simulink model "CerebellumIODCNAbstractFext"  (Simulink 7.4)
settings: Solver=ode3  StartTime=0.0  StopTime=1.  FixedStep=0.002  RelTol=1e-3
values from neighbouring files (symbols this model uses):
  RRedKuKa = RRedKuKa    [LaunchCerebellumSimulink.m]    (also in LaunchCerebellumSimulinkExternalForce.m; MANIPULATORS.mat = )
undefined symbols (not defined in the file or in its folder): frne
libraries: simulink x1
(part 1 of 2)
settings Model: Creator=Sensopac  LastModifiedBy=Sensopac
settings SimEventsCC: propDiagAttribOutput=1  propDiagFcnCallOutput=1  propDiagStatOutput=0

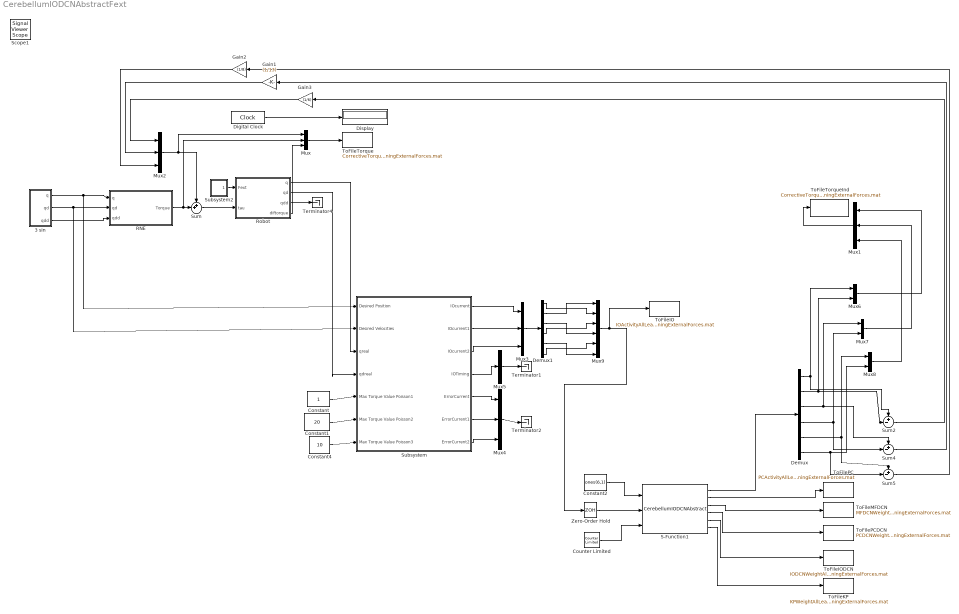
== system CerebellumIODCNAbstractFext ==
  3 sin : Subsystem
  Constant : Constant  OutDataType=sfix(16)  OutScaling=2^0
  Constant1 : Constant  Value=20  OutDataType=sfix(16)  OutScaling=2^0
  Constant2 : Constant  Value=ones(6,1)  OutDataTypeMode=double  OutDataType=sfix(16)  OutScaling=2^0  OutDataTypeStr=double  SampleTime=0.002
  Constant4 : Constant  Value=10  OutDataType=sfix(16)  OutScaling=2^0
  Counter Limited : simulink/Sources/Counter Limited  SystemSampleTime=-1  uplimit=499  tsamp=0.002
  Demux : Demux  Outputs=6
  Demux1 : Demux  Outputs=6
  Digital Clock : DigitalClock  SampleTime=0.002
  Display : Display
  Gain1 : Gain  Gain=(1/13)  ParameterDataType=fixdt(1, 16)  ParameterScaling=2^0  OutDataType=fixdt(1, 16)  OutScaling=2^0
  Gain2 : Gain  Gain=(1/8)  ParameterDataType=fixdt(1, 16)  ParameterScaling=2^0  OutDataType=fixdt(1, 16)  OutScaling=2^0
  Gain3 : Gain  Gain=(1/6)  ParameterDataType=fixdt(1, 16)  ParameterScaling=2^0  OutDataType=fixdt(1, 16)  OutScaling=2^0
  Mux{,1..4} (5 alike) : Mux  Inputs=3
  Mux5 : Mux  Inputs=1
  Mux6 : Mux  Inputs=2
  Mux7 : Mux  Inputs=2
  Mux8 : Mux  Inputs=2
  Mux9 : Mux  Inputs=6
  "RNE " : Subsystem  mask{grav=[ 0 0 9.81], RRed=RRedKuKa}
      mask prompts: grav "Gravity Vector( 0 0  -9.81)"; RRed "Robot"
      mask help:
      | This block computes the inverse dynamics by using the
      | recursive Newton Euler algorithm(computationally speaking more efficient than Lagrange-Euler's method)
      | The gravity vector has to be set (the gravity direction has to be taken into account)
      mask Display:
      | port_label('output',1,'Torques')
      | port_label('input',1,'q')
      | port_label('input',2,'qd')
      | port_label('input',3,'qdd')
      | fprintf('RNE')
  Robot : Subsystem
  S-Function1 : S-Function  FunctionName=CerebellumIODCNAbstract  Parameters=ParamFile NumberOfJoints NumberOfStates WeightFile  EnableBusSupport=off  mask{ParamFile='Parameters.txt', NumberOfJoints=6, NumberOfStates=500, WeightFile='./Register/WeightsNF.dat'}
      mask prompts: ParamFile "Learning Configuration File"; NumberOfJoints "Number Of Joints"; NumberOfStates "Number Of States"; WeightFile "Final Weight File"
      mask Display:
      | image(imread('EDLUTIcon.jpg'));
      | port_label('input',1,'MFAct')
      | port_label('input',2,'Error')
      | port_label('input',3,'State')
      | port_label('output',1,'DCNAct')
      | port_label('output',2,'PCAct')
      | port_label('output',3,'MFWeight')
      | port_label('output',4,'PCWeight')
      | port_label('output',5,'IOWeight')
      | port_label('output',6,'KPWeight')
      | fprintf('Cerebellum')
  Subsystem : Subsystem
  Subsystem2 : Subsystem
  Sum : Sum  Inputs=++|  OutDataType=sfix(16)  OutScaling=2^0
  Sum2 : Sum  Inputs=+-|  OutDataType=sfix(16)  OutScaling=2^0
  Sum4 : Sum  Inputs=+-|  OutDataType=sfix(16)  OutScaling=2^0
  Sum5 : Sum  Inputs=+-|  OutDataType=sfix(16)  OutScaling=2^0
  Terminator1 : Terminator
  Terminator2 : Terminator
  Terminator4 : Terminator
  ToFileIO : ToFile  Filename=IOActivityAllLearningExternalForces.mat
  ToFileIODCN : ToFile  Filename=IODCNWeightAllLearningExternalForces.mat
  ToFileKP : ToFile  Filename=KPWeightAllLearningExternalForces.mat
  ToFileMFDCN : ToFile  Filename=MFDCNWeightAllLearningExternalForces.mat
  ToFilePC : ToFile  Filename=PCActivityAllLearningExternalForces.mat
  ToFilePCDCN : ToFile  Filename=PCDCNWeightAllLearningExternalForces.mat
  ToFileTorque : ToFile  Filename=CorrectiveTorqueAllLearningExternalForces.mat
  ToFileTorqueInd : ToFile  Filename=CorrectiveTorque1AllLearningExternalForces.mat
  Zero-Order Hold : ZeroOrderHold  SampleTime=0.002
  Scope1 : SignalViewerScope  IOType=viewer  RefreshTime=0.035000
  wires:
  3 sin/1(q) -> Subsystem/1(Desired Position), "RNE "/1(q)
  3 sin/2(qd) -> Subsystem/2(Desired Velocities), "RNE "/2(qd)
  3 sin/3(qdd) -> "RNE "/3(qdd)
  "RNE "/1(Torque) -> Sum/2, Mux/2
  Robot/1(q) -> Subsystem/3(qreal)
  Robot/2(qd) -> Subsystem/4(qdreal)
  Sum/1 -> Robot/2(tau)
  Robot/3(qdd) -> Terminator4/1
  Mux2/1 -> Mux/1, Sum/1
  Mux/1 -> ToFileTorque/1
  Mux1/1 -> ToFileTorqueInd/1
  Counter Limited/1 -> S-Function1/3
  Constant2/1 -> S-Function1/1
  S-Function1/1 -> Demux/1
  S-Function1/2 -> ToFilePC/1
  S-Function1/3 -> ToFileMFDCN/1
  S-Function1/4 -> ToFilePCDCN/1
  Zero-Order Hold/1 -> S-Function1/2
  Mux6/1 -> Mux1/1
  Mux7/1 -> Mux1/2
  Mux8/1 -> Mux1/3
  Demux/1 -> Sum2/1, Mux6/1
  Demux/3 -> Sum4/1, Mux7/1
  Demux/5 -> Sum5/1, Mux8/1
  Demux/6 -> Sum5/2, Mux8/2
  Demux/4 -> Sum4/2, Mux7/2
  Demux/2 -> Sum2/2, Mux6/2
  Sum2/1 -> Gain3/1
  Sum4/1 -> Gain1/1
  Sum5/1 -> Gain2/1
  Mux5/1 -> Terminator1/1
  Mux4/1 -> Terminator2/1
  Subsystem/4(IOTiming) -> Mux5/1
  Subsystem/5(ErrorCurrent) -> Mux4/1
  Subsystem/6(ErrorCurrent1) -> Mux4/2
  Subsystem/7(ErrorCurrent2) -> Mux4/3
  Mux3/1 -> Demux1/1
  Mux9/1 -> ToFileIO/1, Zero-Order Hold/1
  Demux1/2 -> Mux9/1
  Demux1/1 -> Mux9/2
  Demux1/3 -> Mux9/4
  Demux1/4 -> Mux9/3
  Demux1/5 -> Mux9/6
  Demux1/6 -> Mux9/5
  Subsystem/1(IOcurrent) -> Mux3/1
  Subsystem/2(IOcurrent1) -> Mux3/2
  Subsystem/3(IOcurrent2) -> Mux3/3
  Digital Clock/1 -> Display/1
  Gain2/1 -> Mux2/3
  Gain1/1 -> Mux2/2
  Gain3/1 -> Mux2/1
  S-Function1/5 -> ToFileIODCN/1
  S-Function1/6 -> ToFileKP/1
  Subsystem2/1(Fx,y,z) -> Robot/1(Fext)
  Robot/4(diftorque) -> Mux/3
  Constant/1 -> Subsystem/5(" Max Torque Value Poisson1")
  Constant1/1 -> Subsystem/6(" Max Torque Value Poisson2")
  Constant4/1 -> Subsystem/7(" Max Torque Value Poisson3")

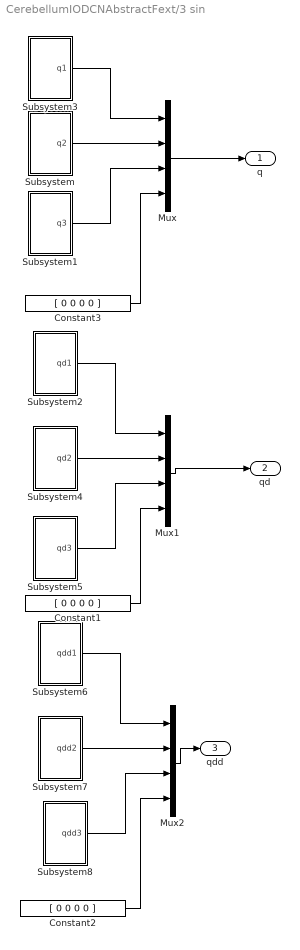
== system CerebellumIODCNAbstractFext/3 sin ==
  Constant1 : Constant  Value=[ 0 0 0 0 ]  OutDataType=sfix(16)  OutScaling=2^0
  Constant2 : Constant  Value=[ 0 0 0 0 ]  OutDataType=sfix(16)  OutScaling=2^0
  Constant3 : Constant  Value=[ 0 0 0 0 ]  OutDataType=sfix(16)  OutScaling=2^0
  Mux : Mux
  Mux1 : Mux
  Mux2 : Mux
  Subsystem : Subsystem
  Subsystem1 : Subsystem
  Subsystem2 : Subsystem
  Subsystem3 : Subsystem
  Subsystem4 : Subsystem
  Subsystem5 : Subsystem
  Subsystem6 : Subsystem
  Subsystem7 : Subsystem
  Subsystem8 : Subsystem
  q : Outport  OutDataType=sfix(16)  OutScaling=2^0
  qd : Outport  Port=2  OutDataType=sfix(16)  OutScaling=2^0
  qdd : Outport  Port=3  OutDataType=sfix(16)  OutScaling=2^0
  wires:
  Mux2/1 -> qdd/1
  Mux1/1 -> qd/1
  Mux/1 -> q/1
  Subsystem3/1(q1) -> Mux/1
  Subsystem/1(q2) -> Mux/2
  Subsystem1/1(q3) -> Mux/3
  Subsystem2/1(qd1) -> Mux1/1
  Subsystem4/1(qd2) -> Mux1/2
  Subsystem5/1(qd3) -> Mux1/3
  Subsystem6/1(qdd1) -> Mux2/1
  Subsystem7/1(qdd2) -> Mux2/2
  Subsystem8/1(qdd3) -> Mux2/3
  Constant3/1 -> Mux/4
  Constant1/1 -> Mux1/4
  Constant2/1 -> Mux2/4

== system CerebellumIODCNAbstractFext/RNE  ==
  q : Inport  OutDataType=sfix(16)  OutScaling=2^0
  qd : Inport  Port=2  OutDataType=sfix(16)  OutScaling=2^0
  qdd : Inport  Port=3  OutDataType=sfix(16)  OutScaling=2^0
  Mux : Mux  Inputs=3
  S-Function : S-Function  FunctionName=Select  Parameters=RRed  EnableBusSupport=off
  S-Function1 : S-Function  FunctionName=Select  Parameters=RRed  EnableBusSupport=off
  S-Function2 : S-Function  FunctionName=Select  Parameters=RRed  EnableBusSupport=off
  rne : MATLABFcn  MATLABFcn=frne(RRed, u(1:RRed.n)', u(RRed.n+1:2*RRed.n)', u(2* RRed.n+1:3*RRed.n)',grav)  OutputDimensions=RRed.n
  Torque : Outport  OutDataType=sfix(16)  OutScaling=2^0
  wires:
  qdd/1 -> S-Function2/1
  rne/1 -> Torque/1
  q/1 -> S-Function/1
  Mux/1 -> rne/1
  qd/1 -> S-Function1/1
  S-Function/1 -> Mux/1
  S-Function1/1 -> Mux/2
  S-Function2/1 -> Mux/3

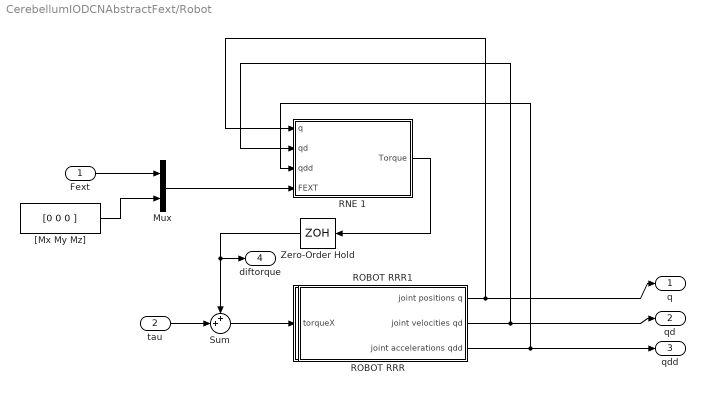
== system CerebellumIODCNAbstractFext/Robot ==
  Fext : Inport  OutDataType=sfix(16)  OutScaling=2^0
  tau : Inport  Port=2  OutDataType=sfix(16)  OutScaling=2^0
  Mux : Mux  Inputs=2
  RNE 1 : Subsystem  mask{grav=[ 0 0 9.81], RRed=RRedKuKa}
      mask prompts: grav "Gravity Vector ( 0 0  -9.81)"; RRed "Robot"
      mask help:
      | This block computes the inverse dynamics by using the
      | recursive Newton Euler algorithm(computationally speaking more efficient than Lagrange-Euler's method)
      | The gravity vector has to be set (the gravity direction has to be taken into account)
      mask Display:
      | port_label('output',1,'Torque')
      | port_label('input',1,'q')
      | port_label('input',2,'qd')
      | port_label('input',3,'qdd')
      | port_label('input',4,'Fext')
      | fprintf('RNE')
  ROBOT RRR : Subsystem  mask{Ciniciales=[0.0  0.1*sin(pi/4)  0.1 0 0 0 0], Viniciales=[2*pi*0.1 2*pi*sin(pi/4)*0.1 0 0 0 0 0], RRed=RRedKuKa}
      mask prompts: Ciniciales "Position initial conditions q"; Viniciales "Velocity initial conditions qd"; RRed "Robot"
      mask help: Simulated robot model(Rigid body dynamics)
  ROBOT RRR1 : Subsystem  mask{Ciniciales=[0.0  0.1*sin(pi/4)  0.1 0 0 0 0], Viniciales=[2*pi*0.1 2*pi*sin(pi/4)*0.1 0 0 0 0 0], RRed=RRedKuKa}
      mask prompts: Ciniciales "Position initial conditions q"; Viniciales "Velocity initial conditions qd"; RRed "Robot"
      mask help: Simulated robot model(Rigid body dynamics)
  Sum : Sum  Inputs=++|  OutDataType=sfix(16)  OutScaling=2^0
  Zero-Order Hold : ZeroOrderHold  SampleTime=0.002
  "[Mx My Mz]" : Constant  Value=[0 0 0 ]  OutDataType=sfix(16)  OutScaling=2^0
  q : Outport  OutDataType=sfix(16)  OutScaling=2^0
  qd : Outport  Port=2  OutDataType=sfix(16)  OutScaling=2^0
  qdd : Outport  Port=3  OutDataType=sfix(16)  OutScaling=2^0
  diftorque : Outport  Port=4  OutDataType=sfix(16)  OutScaling=2^0
  wires:
  ROBOT RRR/1(joint positions q) -> q/1, RNE 1/1(q)
  ROBOT RRR/2(joint velocities qd) -> qd/1, RNE 1/2(qd)
  ROBOT RRR/3(joint accelerations qdd) -> qdd/1, RNE 1/3(qdd)
  tau/1 -> Sum/2
  "[Mx My Mz]"/1 -> Mux/2
  Fext/1 -> Mux/1
  Mux/1 -> RNE 1/4(FEXT)
  RNE 1/1(Torque) -> Zero-Order Hold/1
  Sum/1 -> ROBOT RRR/1(torqueX)
  Zero-Order Hold/1 -> Sum/1, diftorque/1

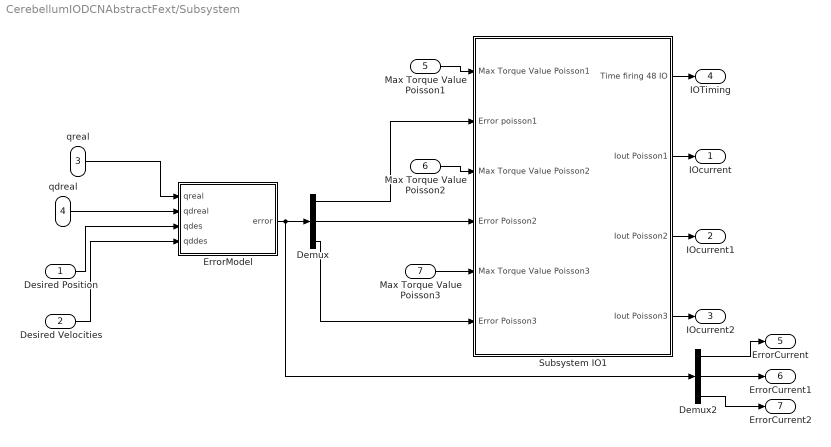
== system CerebellumIODCNAbstractFext/Subsystem ==
  Desired Position : Inport
  Desired Velocities : Inport  Port=2
  qreal : Inport  Port=3  OutDataType=sfix(16)  OutScaling=2^0
  qdreal : Inport  Port=4  OutDataType=sfix(16)  OutScaling=2^0
  " Max Torque Value Poisson1" : Inport  Port=5  OutDataType=sfix(16)  OutScaling=2^0
  " Max Torque Value Poisson2" : Inport  Port=6  OutDataType=sfix(16)  OutScaling=2^0
  " Max Torque Value Poisson3" : Inport  Port=7  OutDataType=sfix(16)  OutScaling=2^0
  Demux : Demux  Outputs=3
  Demux2 : Demux  Outputs=3
  ErrorModel : Subsystem
  Subsystem IO1 : Subsystem
  IOcurrent : Outport
  IOcurrent1 : Outport  Port=2
  IOcurrent2 : Outport  Port=3
  IOTiming : Outport  Port=4
  ErrorCurrent : Outport  Port=5
  ErrorCurrent1 : Outport  Port=6
  ErrorCurrent2 : Outport  Port=7
  wires:
  Desired Position/1 -> ErrorModel/3(qdes)
  Desired Velocities/1 -> ErrorModel/4(qddes)
  Subsystem IO1/1(Time firing 48 IO) -> IOTiming/1
  Demux/1 -> Subsystem IO1/2(Error poisson1)
  Subsystem IO1/2(Iout Poisson1) -> IOcurrent/1
  Demux/2 -> Subsystem IO1/4(Error Poisson2)
  Subsystem IO1/3(Iout Poisson2) -> IOcurrent1/1
  Demux/3 -> Subsystem IO1/6(Error Poisson3)
  Subsystem IO1/4(Iout Poisson3) -> IOcurrent2/1
  ErrorModel/1(error) -> Demux/1, Demux2/1
  qreal/1 -> ErrorModel/1(qreal)
  qdreal/1 -> ErrorModel/2(qdreal)
  Demux2/1 -> ErrorCurrent/1
  Demux2/2 -> ErrorCurrent1/1
  Demux2/3 -> ErrorCurrent2/1
  " Max Torque Value Poisson1"/1 -> Subsystem IO1/1(" Max Torque Value Poisson1")
  " Max Torque Value Poisson2"/1 -> Subsystem IO1/3(" Max Torque Value Poisson2")
  " Max Torque Value Poisson3"/1 -> Subsystem IO1/5(" Max Torque Value Poisson3")

== system CerebellumIODCNAbstractFext/Subsystem2 ==
  Mux : Mux  Inputs=3
  Subsystem : Subsystem
  Subsystem1 : Subsystem
  Subsystem3 : Subsystem
  Fx,y,z : Outport  OutDataType=sfix(16)  OutScaling=2^0
  wires:
  Mux/1 -> Fx,y,z/1
  Subsystem3/1(q1) -> Mux/1
  Subsystem/1(q2) -> Mux/2
  Subsystem1/1(q3) -> Mux/3

== system CerebellumIODCNAbstractFext/3 sin/Subsystem ==
  Constant1 : Constant  Value=0.1  OutDataType=sfix(16)  OutScaling=2^0
  Constant2 : Constant  Value=pi/4  OutDataType=sfix(16)  OutScaling=2^0
  Constant3 : Constant  Value=2*pi  OutDataType=sfix(16)  OutScaling=2^0
  Digital Clock : DigitalClock  SampleTime=0.002
  Product : Product  OutDataType=sfix(16)  OutScaling=2^0  RndMeth=Zero
  Product2 : Product  OutDataType=sfix(16)  OutScaling=2^0  RndMeth=Zero
  Sum : Sum  Inputs=|++  OutDataType=sfix(16)  OutScaling=2^0
  Trigonometric Function : Trigonometry
  q2 : Outport  OutDataType=sfix(16)  OutScaling=2^0
  wires:
  Sum/1 -> Trigonometric Function/1
  Constant2/1 -> Sum/1
  Product2/1 -> Sum/2
  Product/1 -> q2/1
  Trigonometric Function/1 -> Product/2
  Constant3/1 -> Product2/1
  Digital Clock/1 -> Product2/2
  Constant1/1 -> Product/1

== system CerebellumIODCNAbstractFext/3 sin/Subsystem1 ==
  Constant2 : Constant  Value=0.1  OutDataType=sfix(16)  OutScaling=2^0
  Constant3 : Constant  Value=pi/2  OutDataType=sfix(16)  OutScaling=2^0
  Constant4 : Constant  Value=2*pi  OutDataType=sfix(16)  OutScaling=2^0
  Digital Clock : DigitalClock  SampleTime=0.002
  Product : Product  OutDataType=sfix(16)  OutScaling=2^0  RndMeth=Zero
  Product2 : Product  OutDataType=sfix(16)  OutScaling=2^0  RndMeth=Zero
  Sum : Sum  Inputs=|++  OutDataType=sfix(16)  OutScaling=2^0
  Trigonometric Function : Trigonometry
  q3 : Outport  OutDataType=sfix(16)  OutScaling=2^0
  wires:
  Sum/1 -> Trigonometric Function/1
  Constant3/1 -> Sum/1
  Product2/1 -> Sum/2
  Product/1 -> q3/1
  Trigonometric Function/1 -> Product/2
  Constant4/1 -> Product2/1
  Digital Clock/1 -> Product2/2
  Constant2/1 -> Product/1

== system CerebellumIODCNAbstractFext/3 sin/Subsystem2 ==
  Constant1 : Constant  Value=0.1*2*pi  OutDataType=sfix(16)  OutScaling=2^0
  Constant3 : Constant  Value=2*pi  OutDataType=sfix(16)  OutScaling=2^0
  Digital Clock : DigitalClock  SampleTime=0.002
  Product : Product  OutDataType=sfix(16)  OutScaling=2^0  RndMeth=Zero
  Product2 : Product  OutDataType=sfix(16)  OutScaling=2^0  RndMeth=Zero
  Trigonometric Function : Trigonometry  Operator=cos
  qd1 : Outport  OutDataType=sfix(16)  OutScaling=2^0
  wires:
  Product/1 -> qd1/1
  Trigonometric Function/1 -> Product/2
  Constant3/1 -> Product2/1
  Product2/1 -> Trigonometric Function/1
  Digital Clock/1 -> Product2/2
  Constant1/1 -> Product/1

== system CerebellumIODCNAbstractFext/3 sin/Subsystem3 ==
  Constant1 : Constant  Value=0.1  OutDataType=sfix(16)  OutScaling=2^0
  Constant3 : Constant  Value=2*pi  OutDataType=sfix(16)  OutScaling=2^0
  Digital Clock : DigitalClock  SampleTime=0.002
  Product : Product  OutDataType=sfix(16)  OutScaling=2^0  RndMeth=Zero
  Product2 : Product  OutDataType=sfix(16)  OutScaling=2^0  RndMeth=Zero
  Trigonometric Function : Trigonometry
  q1 : Outport  OutDataType=sfix(16)  OutScaling=2^0
  wires:
  Product/1 -> q1/1
  Trigonometric Function/1 -> Product/2
  Constant3/1 -> Product2/1
  Product2/1 -> Trigonometric Function/1
  Digital Clock/1 -> Product2/2
  Constant1/1 -> Product/1

== system CerebellumIODCNAbstractFext/3 sin/Subsystem4 ==
  Constant1 : Constant  Value=0.1*2*pi  OutDataType=sfix(16)  OutScaling=2^0
  Constant2 : Constant  Value=pi/4  OutDataType=sfix(16)  OutScaling=2^0
  Constant3 : Constant  Value=2*pi  OutDataType=sfix(16)  OutScaling=2^0
  Digital Clock : DigitalClock  SampleTime=0.002
  Product : Product  OutDataType=sfix(16)  OutScaling=2^0  RndMeth=Zero
  Product2 : Product  OutDataType=sfix(16)  OutScaling=2^0  RndMeth=Zero
  Sum : Sum  Inputs=|++  OutDataType=sfix(16)  OutScaling=2^0
  Trigonometric Function : Trigonometry  Operator=cos
  qd2 : Outport  OutDataType=sfix(16)  OutScaling=2^0
  wires:
  Sum/1 -> Trigonometric Function/1
  Constant2/1 -> Sum/1
  Product2/1 -> Sum/2
  Product/1 -> qd2/1
  Trigonometric Function/1 -> Product/2
  Constant3/1 -> Product2/1
  Digital Clock/1 -> Product2/2
  Constant1/1 -> Product/1

== system CerebellumIODCNAbstractFext/3 sin/Subsystem5 ==
  Constant1 : Constant  Value=0.1*2*pi  OutDataType=sfix(16)  OutScaling=2^0
  Constant3 : Constant  Value=pi/2  OutDataType=sfix(16)  OutScaling=2^0
  Constant4 : Constant  Value=2*pi  OutDataType=sfix(16)  OutScaling=2^0
  Digital Clock : DigitalClock  SampleTime=0.002
  Product : Product  OutDataType=sfix(16)  OutScaling=2^0  RndMeth=Zero
  Product2 : Product  OutDataType=sfix(16)  OutScaling=2^0  RndMeth=Zero
  Sum : Sum  Inputs=|++  OutDataType=sfix(16)  OutScaling=2^0
  Trigonometric Function : Trigonometry  Operator=cos
  qd3 : Outport  OutDataType=sfix(16)  OutScaling=2^0
  wires:
  Sum/1 -> Trigonometric Function/1
  Constant3/1 -> Sum/1
  Product2/1 -> Sum/2
  Product/1 -> qd3/1
  Trigonometric Function/1 -> Product/2
  Constant4/1 -> Product2/1
  Digital Clock/1 -> Product2/2
  Constant1/1 -> Product/1

== system CerebellumIODCNAbstractFext/3 sin/Subsystem6 ==
  Constant1 : Constant  Value=-0.1*4*pi^2  OutDataType=sfix(16)  OutScaling=2^0
  Constant3 : Constant  Value=2*pi  OutDataType=sfix(16)  OutScaling=2^0
  Digital Clock : DigitalClock  SampleTime=0.002
  Product : Product  OutDataType=sfix(16)  OutScaling=2^0  RndMeth=Zero
  Product2 : Product  OutDataType=sfix(16)  OutScaling=2^0  RndMeth=Zero
  Trigonometric Function : Trigonometry
  qdd1 : Outport  OutDataType=sfix(16)  OutScaling=2^0
  wires:
  Product/1 -> qdd1/1
  Trigonometric Function/1 -> Product/2
  Constant3/1 -> Product2/1
  Product2/1 -> Trigonometric Function/1
  Digital Clock/1 -> Product2/2
  Constant1/1 -> Product/1

== system CerebellumIODCNAbstractFext/3 sin/Subsystem7 ==
  Constant1 : Constant  Value=-0.1*4*pi^2  OutDataType=sfix(16)  OutScaling=2^0
  Constant2 : Constant  Value=pi/4  OutDataType=sfix(16)  OutScaling=2^0
  Constant3 : Constant  Value=2*pi  OutDataType=sfix(16)  OutScaling=2^0
  Digital Clock : DigitalClock  SampleTime=0.002
  Product : Product  OutDataType=sfix(16)  OutScaling=2^0  RndMeth=Zero
  Product2 : Product  OutDataType=sfix(16)  OutScaling=2^0  RndMeth=Zero
  Sum : Sum  Inputs=|++  OutDataType=sfix(16)  OutScaling=2^0
  Trigonometric Function : Trigonometry
  qdd2 : Outport  OutDataType=sfix(16)  OutScaling=2^0
  wires:
  Sum/1 -> Trigonometric Function/1
  Constant2/1 -> Sum/1
  Product2/1 -> Sum/2
  Product/1 -> qdd2/1
  Trigonometric Function/1 -> Product/2
  Constant3/1 -> Product2/1
  Digital Clock/1 -> Product2/2
  Constant1/1 -> Product/1

== system CerebellumIODCNAbstractFext/3 sin/Subsystem8 ==
  Constant1 : Constant  Value=-0.1*4*pi^2  OutDataType=sfix(16)  OutScaling=2^0
  Constant3 : Constant  Value=pi/2  OutDataType=sfix(16)  OutScaling=2^0
  Constant4 : Constant  Value=2*pi  OutDataType=sfix(16)  OutScaling=2^0
  Digital Clock : DigitalClock  SampleTime=0.002
  Product : Product  OutDataType=sfix(16)  OutScaling=2^0  RndMeth=Zero
  Product2 : Product  OutDataType=sfix(16)  OutScaling=2^0  RndMeth=Zero
  Sum : Sum  Inputs=|++  OutDataType=sfix(16)  OutScaling=2^0
  Trigonometric Function : Trigonometry
  qdd3 : Outport  OutDataType=sfix(16)  OutScaling=2^0
  wires:
  Sum/1 -> Trigonometric Function/1
  Constant3/1 -> Sum/1
  Product2/1 -> Sum/2
  Product/1 -> qdd3/1
  Trigonometric Function/1 -> Product/2
  Constant4/1 -> Product2/1
  Digital Clock/1 -> Product2/2
  Constant1/1 -> Product/1

== system CerebellumIODCNAbstractFext/Robot/RNE 1 ==
  q : Inport  OutDataType=sfix(16)  OutScaling=2^0
  qd : Inport  Port=2  OutDataType=sfix(16)  OutScaling=2^0
  qdd : Inport  Port=3  OutDataType=sfix(16)  OutScaling=2^0
  FEXT : Inport  Port=4  OutDataType=sfix(16)  OutScaling=2^0
  Mux : Mux
  rne : MATLABFcn  MATLABFcn=frne(RRed, u(1:RRed.n)', u(RRed.n+1:2*RRed.n)', u(2* RRed.n+1:3*RRed.n)',grav,u(3*RRed.n+1:end)')-frne(RRed, u(1:RRed.n)', u(RRed.n+1:2*RRed.n)', u(2* RRed.n+1:3*RRed.n)',grav)  OutputDimensions=RRed.n
  Torque : Outport  OutDataType=sfix(16)  OutScaling=2^0
  wires:
  FEXT/1 -> Mux/4
  qdd/1 -> Mux/3
  qd/1 -> Mux/2
  q/1 -> Mux/1
  Mux/1 -> rne/1
  rne/1 -> Torque/1

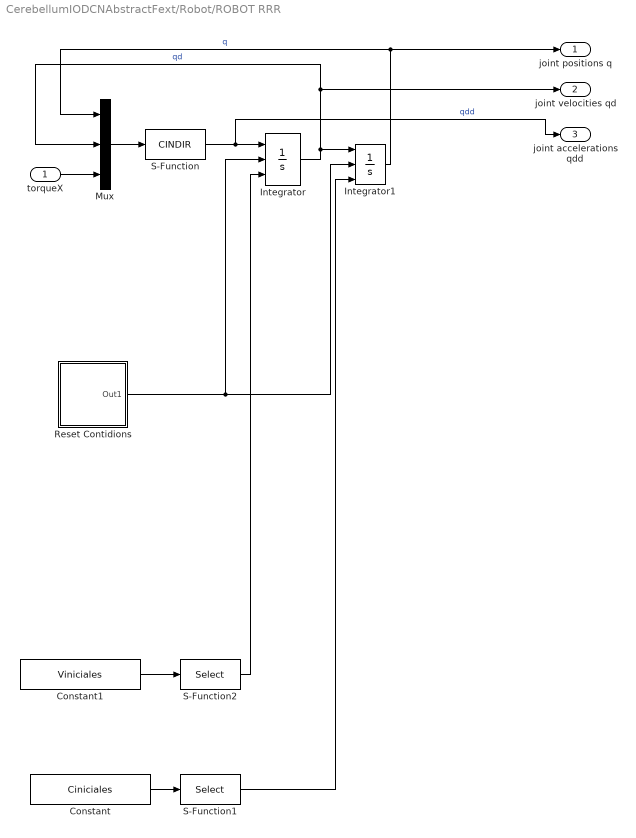
== system CerebellumIODCNAbstractFext/Robot/ROBOT RRR ==
  torqueX : Inport  OutDataType=sfix(16)  OutScaling=2^0
  Constant : Constant  Value=Ciniciales  OutDataType=sfix(16)  OutScaling=2^0
  Constant1 : Constant  Value=Viniciales  OutDataType=sfix(16)  OutScaling=2^0
  Integrator : Integrator  ExternalReset=falling  InitialConditionSource=external
  Integrator1 : Integrator  ExternalReset=falling  InitialConditionSource=external
  Mux : Mux  Inputs=3
  Reset Contidions : Subsystem  mask{T=1}
      mask prompts: T "Period"
      mask Display: port_label ('output',1,'FallingReset')
  S-Function : S-Function  FunctionName=CINDIR  Parameters=RRed  EnableBusSupport=off
  S-Function1 : S-Function  FunctionName=Select  Parameters=RRed  EnableBusSupport=off
  S-Function2 : S-Function  FunctionName=Select  Parameters=RRed  EnableBusSupport=off
  joint positions q : Outport  OutDataType=sfix(16)  OutScaling=2^0
  joint velocities qd : Outport  Port=2  OutDataType=sfix(16)  OutScaling=2^0
  joint accelerations qdd : Outport  Port=3  OutDataType=sfix(16)  OutScaling=2^0
  wires:
  torqueX/1 -> Mux/3
  Integrator/1 -> Integrator1/1, Mux/2, joint velocities qd/1  "qd"
  Mux/1 -> S-Function/1
  S-Function/1 -> Integrator/1, joint accelerations qdd/1  "qdd"
  Constant/1 -> S-Function1/1
  Integrator1/1 -> Mux/1, joint positions q/1  "q"
  S-Function1/1 -> Integrator1/3
  S-Function2/1 -> Integrator/3
  Constant1/1 -> S-Function2/1
  Reset Contidions/1(Out1) -> Integrator1/2, Integrator/2

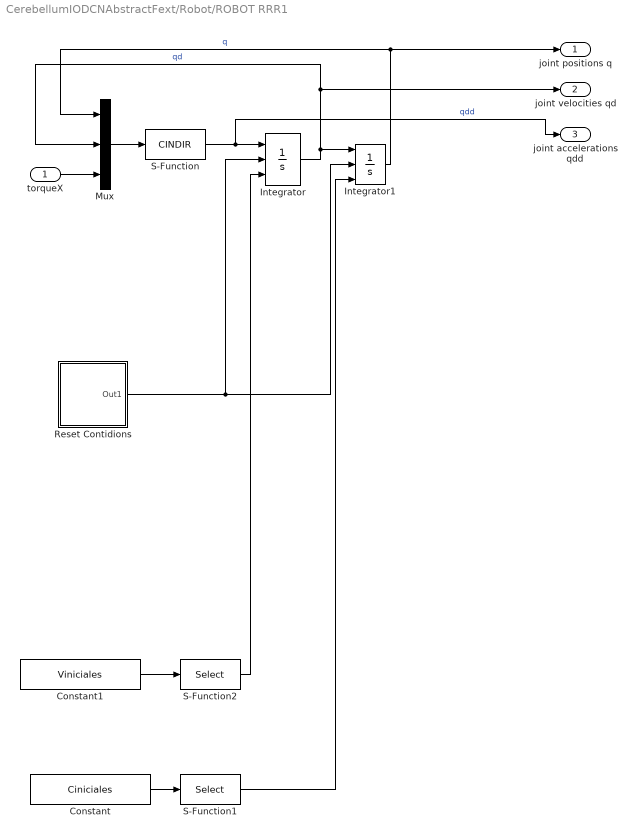
== system CerebellumIODCNAbstractFext/Robot/ROBOT RRR1 ==
  torqueX : Inport  OutDataType=sfix(16)  OutScaling=2^0
  Constant : Constant  Value=Ciniciales  OutDataType=sfix(16)  OutScaling=2^0
  Constant1 : Constant  Value=Viniciales  OutDataType=sfix(16)  OutScaling=2^0
  Integrator : Integrator  ExternalReset=falling  InitialConditionSource=external
  Integrator1 : Integrator  ExternalReset=falling  InitialConditionSource=external
  Mux : Mux  Inputs=3
  Reset Contidions : Subsystem  mask{T=1}
      mask prompts: T "Period"
      mask Display: port_label ('output',1,'FallingReset')
  S-Function : S-Function  FunctionName=CINDIR  Parameters=RRed  EnableBusSupport=off
  S-Function1 : S-Function  FunctionName=Select  Parameters=RRed  EnableBusSupport=off
  S-Function2 : S-Function  FunctionName=Select  Parameters=RRed  EnableBusSupport=off
  joint positions q : Outport  OutDataType=sfix(16)  OutScaling=2^0
  joint velocities qd : Outport  Port=2  OutDataType=sfix(16)  OutScaling=2^0
  joint accelerations qdd : Outport  Port=3  OutDataType=sfix(16)  OutScaling=2^0
  wires:
  Reset Contidions/1(Out1) -> Integrator/2, Integrator1/2
  Constant1/1 -> S-Function2/1
  S-Function2/1 -> Integrator/3
  S-Function1/1 -> Integrator1/3
  Integrator1/1 -> joint positions q/1, Mux/1  "q"
  Constant/1 -> S-Function1/1
  S-Function/1 -> joint accelerations qdd/1, Integrator/1  "qdd"
  Mux/1 -> S-Function/1
  Integrator/1 -> joint velocities qd/1, Mux/2, Integrator1/1  "qd"
  torqueX/1 -> Mux/3

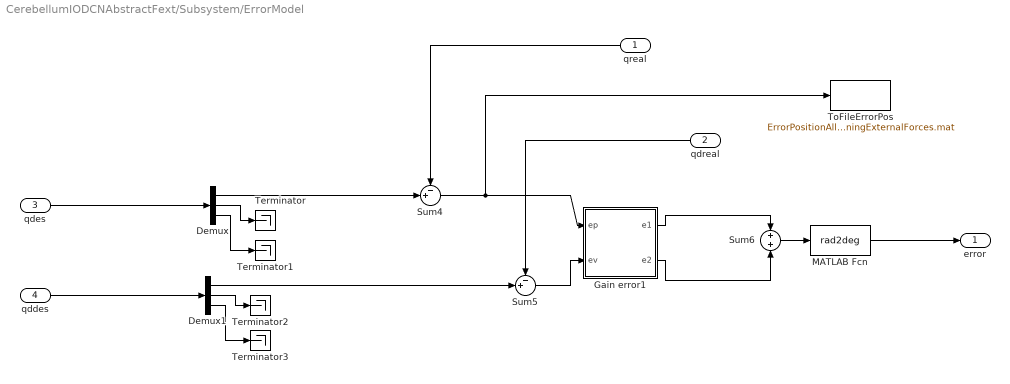
== system CerebellumIODCNAbstractFext/Subsystem/ErrorModel ==
  qreal : Inport  OutDataType=sfix(16)  OutScaling=2^0
  qdreal : Inport  Port=2  OutDataType=sfix(16)  OutScaling=2^0
  qdes : Inport  Port=3  OutDataType=sfix(16)  OutScaling=2^0
  qddes : Inport  Port=4  OutDataType=sfix(16)  OutScaling=2^0
  Demux : Demux  Outputs=3
  Demux1 : Demux  Outputs=3
  Gain error1 : Subsystem  mask{KP1=2, KP2=10, KP3=6, KV1=0.2, KV2=10*0.1, KV3=0.6}
      mask prompts: KP1 "Error Position Gain Value 1"; KP2 "Error Position Gain Value 2"; KP3 "Error Position Gain Value3"; KV1 "Error Velocity Gain Value1"; KV2 "Error Velocity Gain Value2"; KV3 "Error Velocity Gain Value3"
  MATLAB Fcn : MATLABFcn  MATLABFcn=rad2deg
  Sum4 : Sum  Inputs=-+|  OutDataType=sfix(16)  OutScaling=2^0
  Sum5 : Sum  Inputs=-+|  OutDataType=sfix(16)  OutScaling=2^0
  Sum6 : Sum  OutDataType=sfix(16)  OutScaling=2^0
  Terminator{,1..3} (4 alike) : Terminator
  ToFileErrorPos : ToFile  Filename=ErrorPositionAllLearningExternalForces.mat
  error : Outport  OutDataType=sfix(16)  OutScaling=2^0
  wires:
  Sum4/1 -> ToFileErrorPos/1, Gain error1/1(ep)
  Sum5/1 -> Gain error1/2(ev)
  Gain error1/1(e1) -> Sum6/1
  Gain error1/2(e2) -> Sum6/2
  qreal/1 -> Sum4/1
  qdreal/1 -> Sum5/1
  qdes/1 -> Demux/1
  qddes/1 -> Demux1/1
  Sum6/1 -> MATLAB Fcn/1
  Demux/1 -> Sum4/2
  Demux1/1 -> Sum5/2
  Demux/2 -> Terminator/1
  Demux/3 -> Terminator1/1
  Demux1/2 -> Terminator2/1
  Demux1/3 -> Terminator3/1
  MATLAB Fcn/1 -> error/1

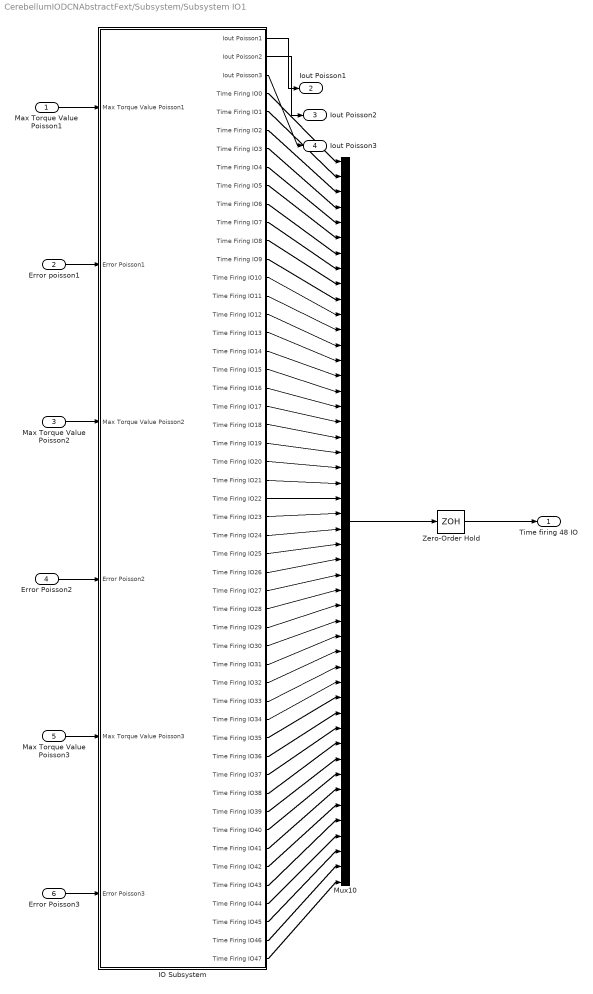
== system CerebellumIODCNAbstractFext/Subsystem/Subsystem IO1 ==
  " Max Torque Value Poisson1" : Inport  OutDataType=sfix(16)  OutScaling=2^0
  Error poisson1 : Inport  Port=2  OutDataType=sfix(16)  OutScaling=2^0
  " Max Torque Value Poisson2" : Inport  Port=3  OutDataType=sfix(16)  OutScaling=2^0
  Error Poisson2 : Inport  Port=4  OutDataType=sfix(16)  OutScaling=2^0
  " Max Torque Value Poisson3" : Inport  Port=5  OutDataType=sfix(16)  OutScaling=2^0
  Error Poisson3 : Inport  Port=6  OutDataType=sfix(16)  OutScaling=2^0
  "IO Subsystem " : Subsystem
  Mux10 : Mux  Inputs=48
  Zero-Order Hold : ZeroOrderHold  SampleTime=0.002
  Time firing 48 IO : Outport  OutDataType=sfix(16)  OutScaling=2^0
  Iout Poisson1 : Outport  Port=2  OutDataType=sfix(16)  OutScaling=2^0
  Iout Poisson2 : Outport  Port=3  OutDataType=sfix(16)  OutScaling=2^0
  Iout Poisson3 : Outport  Port=4  OutDataType=sfix(16)  OutScaling=2^0
  wires:
  " Max Torque Value Poisson1"/1 -> "IO Subsystem "/1(" Max Torque Value Poisson1")
  Error poisson1/1 -> "IO Subsystem "/2(Error Poisson1)
  " Max Torque Value Poisson2"/1 -> "IO Subsystem "/3(" Max Torque Value Poisson2")
  Error Poisson2/1 -> "IO Subsystem "/4(Error Poisson2)
  "IO Subsystem "/1(Iout Poisson1) -> Iout Poisson1/1
  "IO Subsystem "/2(Iout Poisson2) -> Iout Poisson2/1
  "IO Subsystem "/3(Iout Poisson3) -> Iout Poisson3/1
  " Max Torque Value Poisson3"/1 -> "IO Subsystem "/5(" Max Torque Value Poisson3")
  Error Poisson3/1 -> "IO Subsystem "/6(Error Poisson3)
  "IO Subsystem "/51(Time Firing IO47) -> Mux10/48
  "IO Subsystem "/4(Time Firing IO0) -> Mux10/1
  "IO Subsystem "/5(Time Firing IO1) -> Mux10/2
  "IO Subsystem "/6(Time Firing IO2) -> Mux10/3
  "IO Subsystem "/7(Time Firing IO3) -> Mux10/4
  "IO Subsystem "/8(Time Firing IO4) -> Mux10/5
  "IO Subsystem "/9(Time Firing IO5) -> Mux10/6
  "IO Subsystem "/10(Time Firing IO6) -> Mux10/7
  "IO Subsystem "/11(Time Firing IO7) -> Mux10/8
  "IO Subsystem "/12(Time Firing IO8) -> Mux10/9
  "IO Subsystem "/13(Time Firing IO9) -> Mux10/10
  "IO Subsystem "/14(Time Firing IO10) -> Mux10/11
  "IO Subsystem "/15(Time Firing IO11) -> Mux10/12
  "IO Subsystem "/16(Time Firing IO12) -> Mux10/13
  "IO Subsystem "/17(Time Firing IO13) -> Mux10/14
  "IO Subsystem "/18(Time Firing IO14) -> Mux10/15
  "IO Subsystem "/19(Time Firing IO15) -> Mux10/16
  "IO Subsystem "/20(Time Firing IO16) -> Mux10/17
  "IO Subsystem "/21(Time Firing IO17) -> Mux10/18
  "IO Subsystem "/22(Time Firing IO18) -> Mux10/19
  "IO Subsystem "/23(Time Firing IO19) -> Mux10/20
  "IO Subsystem "/24(Time Firing IO20) -> Mux10/21
  "IO Subsystem "/50(Time Firing IO46) -> Mux10/47
  "IO Subsystem "/49(Time Firing IO45) -> Mux10/46
  "IO Subsystem "/48(Time Firing IO44) -> Mux10/45
  "IO Subsystem "/47(Time Firing IO43) -> Mux10/44
  "IO Subsystem "/46(Time Firing IO42) -> Mux10/43
  "IO Subsystem "/45(Time Firing IO41) -> Mux10/42
  "IO Subsystem "/44(Time Firing IO40) -> Mux10/41
  "IO Subsystem "/43(Time Firing IO39) -> Mux10/40
  "IO Subsystem "/42(Time Firing IO38) -> Mux10/39
  "IO Subsystem "/41(Time Firing IO37) -> Mux10/38
  "IO Subsystem "/40(Time Firing IO36) -> Mux10/37
  "IO Subsystem "/39(Time Firing IO35) -> Mux10/36
  "IO Subsystem "/38(Time Firing IO34) -> Mux10/35
  "IO Subsystem "/37(Time Firing IO33) -> Mux10/34
  "IO Subsystem "/36(Time Firing IO32) -> Mux10/33
  "IO Subsystem "/35(Time Firing IO31) -> Mux10/32
  "IO Subsystem "/34(Time Firing IO30) -> Mux10/31
  "IO Subsystem "/32(Time Firing IO28) -> Mux10/29
  "IO Subsystem "/33(Time Firing IO29) -> Mux10/30
  "IO Subsystem "/31(Time Firing IO27) -> Mux10/28
  "IO Subsystem "/30(Time Firing IO26) -> Mux10/27
  "IO Subsystem "/29(Time Firing IO25) -> Mux10/26
  "IO Subsystem "/28(Time Firing IO24) -> Mux10/25
  "IO Subsystem "/27(Time Firing IO23) -> Mux10/24
  "IO Subsystem "/26(Time Firing IO22) -> Mux10/23
  "IO Subsystem "/25(Time Firing IO21) -> Mux10/22
  Mux10/1 -> Zero-Order Hold/1
  Zero-Order Hold/1 -> Time firing 48 IO/1

== system CerebellumIODCNAbstractFext/Subsystem2/Subsystem ==
  Constant1 : Constant  Value=100  OutDataType=sfix(16)  OutScaling=2^0
  Constant2 : Constant  Value=pi/4  OutDataType=sfix(16)  OutScaling=2^0
  Constant3 : Constant  Value=20*pi  OutDataType=sfix(16)  OutScaling=2^0
  Digital Clock : DigitalClock  SampleTime=0.002
  Product : Product  OutDataType=sfix(16)  OutScaling=2^0  RndMeth=Zero
  Product2 : Product  OutDataType=sfix(16)  OutScaling=2^0  RndMeth=Zero
  Sum : Sum  Inputs=|++  OutDataType=sfix(16)  OutScaling=2^0
  Trigonometric Function : Trigonometry  Operator=cos
  q2 : Outport  OutDataType=sfix(16)  OutScaling=2^0
  wires:
  Sum/1 -> Trigonometric Function/1
  Constant2/1 -> Sum/1
  Product2/1 -> Sum/2
  Product/1 -> q2/1
  Trigonometric Function/1 -> Product/2
  Constant3/1 -> Product2/1
  Digital Clock/1 -> Product2/2
  Constant1/1 -> Product/1

== system CerebellumIODCNAbstractFext/Subsystem2/Subsystem1 ==
  Constant2 : Constant  Value=100  OutDataType=sfix(16)  OutScaling=2^0
  Constant3 : Constant  Value=pi/2  OutDataType=sfix(16)  OutScaling=2^0
  Constant4 : Constant  Value=20*pi  OutDataType=sfix(16)  OutScaling=2^0
  Digital Clock : DigitalClock  SampleTime=0.002
  Product : Product  OutDataType=sfix(16)  OutScaling=2^0  RndMeth=Zero
  Product2 : Product  OutDataType=sfix(16)  OutScaling=2^0  RndMeth=Zero
  Sum : Sum  Inputs=|++  OutDataType=sfix(16)  OutScaling=2^0
  Trigonometric Function : Trigonometry  Operator=cos
  q3 : Outport  OutDataType=sfix(16)  OutScaling=2^0
  wires:
  Sum/1 -> Trigonometric Function/1
  Constant3/1 -> Sum/1
  Product2/1 -> Sum/2
  Product/1 -> q3/1
  Trigonometric Function/1 -> Product/2
  Constant4/1 -> Product2/1
  Digital Clock/1 -> Product2/2
  Constant2/1 -> Product/1

== system CerebellumIODCNAbstractFext/Subsystem2/Subsystem3 ==
  Constant1 : Constant  Value=100  OutDataType=sfix(16)  OutScaling=2^0
  Constant3 : Constant  Value=20*pi  OutDataType=sfix(16)  OutScaling=2^0
  Digital Clock : DigitalClock  SampleTime=0.002
  Product : Product  OutDataType=sfix(16)  OutScaling=2^0  RndMeth=Zero
  Product2 : Product  OutDataType=sfix(16)  OutScaling=2^0  RndMeth=Zero
  Trigonometric Function : Trigonometry  Operator=cos
  q1 : Outport  OutDataType=sfix(16)  OutScaling=2^0
  wires:
  Product/1 -> q1/1
  Trigonometric Function/1 -> Product/2
  Constant3/1 -> Product2/1
  Product2/1 -> Trigonometric Function/1
  Digital Clock/1 -> Product2/2
  Constant1/1 -> Product/1

== system CerebellumIODCNAbstractFext/Robot/ROBOT RRR/Reset Contidions ==
  Constant2 : Constant  Value=T  OutDataType=fixdt(1, 16)  OutScaling=2^0
  Digital Clock : DigitalClock  SampleTime=0.002
  Math Function : Math  Operator=mod  OutputSignalType=real  OutDataType=fixdt(1, 16)  OutScaling=2^0  SaturateOnIntegerOverflow=on
  Out1 : Outport
  wires:
  Digital Clock/1 -> Math Function/1
  Constant2/1 -> Math Function/2
  Math Function/1 -> Out1/1

== system CerebellumIODCNAbstractFext/Robot/ROBOT RRR1/Reset Contidions ==
  Constant2 : Constant  Value=T  OutDataType=fixdt(1, 16)  OutScaling=2^0
  Digital Clock : DigitalClock  SampleTime=0.002
  Math Function : Math  Operator=mod  OutputSignalType=real  OutDataType=fixdt(1, 16)  OutScaling=2^0  SaturateOnIntegerOverflow=on
  Out1 : Outport
  wires:
  Math Function/1 -> Out1/1
  Constant2/1 -> Math Function/2
  Digital Clock/1 -> Math Function/1

== system CerebellumIODCNAbstractFext/Subsystem/ErrorModel/Gain error1 ==
  ep : Inport  OutDataType=sfix(16)  OutScaling=2^0
  ev : Inport  Port=2  OutDataType=sfix(16)  OutScaling=2^0
  Gain : Gain  Gain=[KP1 0 0;0 KP2 0;0 0 KP3]  Multiplication=Matrix(K*u)  ParameterDataType=sfix(16)  ParameterScaling=2^0  OutDataType=sfix(16)  OutScaling=2^0
  Gain1 : Gain  Gain=[KV1 0 0;0 KV2 0; 0 0 KV3]  Multiplication=Matrix(K*u)  ParameterDataType=sfix(16)  ParameterScaling=2^0  OutDataType=sfix(16)  OutScaling=2^0
  e1 : Outport  OutDataType=sfix(16)  OutScaling=2^0
  e2 : Outport  Port=2  OutDataType=sfix(16)  OutScaling=2^0
  wires:
  ep/1 -> Gain/1
  ev/1 -> Gain1/1
  Gain/1 -> e1/1
  Gain1/1 -> e2/1

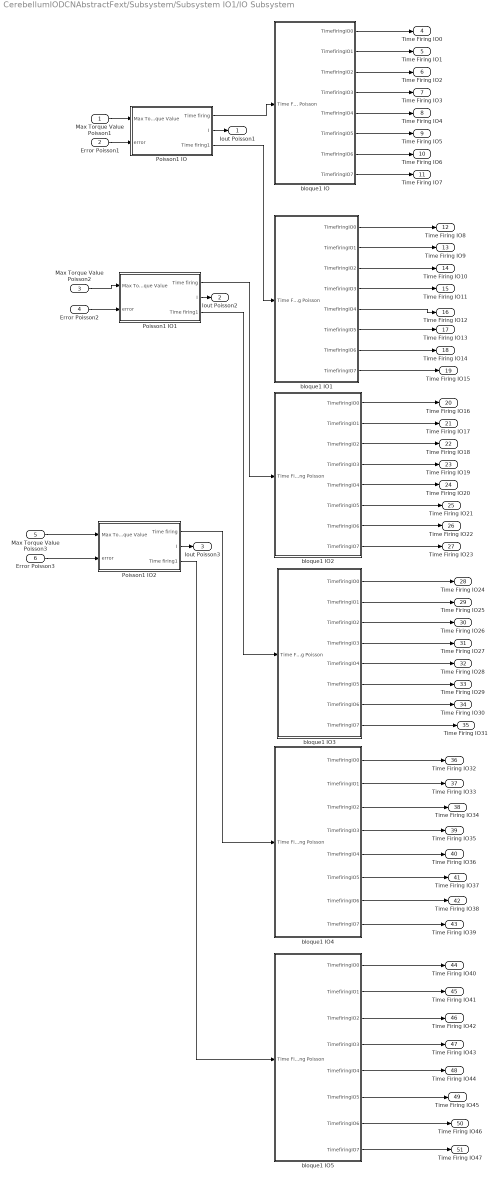
== system CerebellumIODCNAbstractFext/Subsystem/Subsystem IO1/IO Subsystem  ==
  " Max Torque Value Poisson1" : Inport  OutDataType=sfix(16)  OutScaling=2^0
  Error Poisson1 : Inport  Port=2  OutDataType=sfix(16)  OutScaling=2^0
  " Max Torque Value Poisson2" : Inport  Port=3  OutDataType=sfix(16)  OutScaling=2^0
  Error Poisson2 : Inport  Port=4  OutDataType=sfix(16)  OutScaling=2^0
  " Max Torque Value Poisson3" : Inport  Port=5  OutDataType=sfix(16)  OutScaling=2^0
  Error Poisson3 : Inport  Port=6  OutDataType=sfix(16)  OutScaling=2^0
  Poisson1 IO : Subsystem  mask{a=0.001, b=1, timestep=0.002, firingrate=50}
      mask prompts: a "A Interval value  [a b] to generate the Poisson distribution"; b "B Interval value  [a b] to generate the Poisson distribution"; timestep "Time Step"
  Poisson1 IO1 : Subsystem  mask{a=0.001, b=1, timestep=0.002, firingrate=50}
      mask prompts: a "A Interval value  [a b] to generate the Poisson distribution"; b "B Interval value  [a b] to generate the Poisson distribution"; timestep "Time Step"
  Poisson1 IO2 : Subsystem  mask{a=0.001, b=1, timestep=0.002, firingrate=50}
      mask prompts: a "A Interval value  [a b] to generate the Poisson distribution"; b "B Interval value  [a b] to generate the Poisson distribution"; timestep "Time Step"
  bloque1 IO : Subsystem
  bloque1 IO1 : Subsystem
  bloque1 IO2 : Subsystem
  bloque1 IO3 : Subsystem
  bloque1 IO4 : Subsystem
  bloque1 IO5 : Subsystem
  Iout Poisson1 : Outport  OutDataType=sfix(16)  OutScaling=2^0
  Iout Poisson2 : Outport  Port=2  OutDataType=sfix(16)  OutScaling=2^0
  Iout Poisson3 : Outport  Port=3  OutDataType=sfix(16)  OutScaling=2^0
  Time Firing IO0 : Outport  Port=4  OutDataType=sfix(16)  OutScaling=2^0
  Time Firing IO1 : Outport  Port=5  OutDataType=sfix(16)  OutScaling=2^0
  Time Firing IO2 : Outport  Port=6  OutDataType=sfix(16)  OutScaling=2^0
  Time Firing IO3 : Outport  Port=7  OutDataType=sfix(16)  OutScaling=2^0
  Time Firing IO4 : Outport  Port=8  OutDataType=sfix(16)  OutScaling=2^0
  Time Firing IO5 : Outport  Port=9  OutDataType=sfix(16)  OutScaling=2^0
  Time Firing IO6 : Outport  Port=10  OutDataType=sfix(16)  OutScaling=2^0
  Time Firing IO7 : Outport  Port=11  OutDataType=sfix(16)  OutScaling=2^0
  Time Firing IO8 : Outport  Port=12  OutDataType=sfix(16)  OutScaling=2^0
  Time Firing IO9 : Outport  Port=13  OutDataType=sfix(16)  OutScaling=2^0
  Time Firing IO10 : Outport  Port=14  OutDataType=sfix(16)  OutScaling=2^0
  Time Firing IO11 : Outport  Port=15  OutDataType=sfix(16)  OutScaling=2^0
  Time Firing IO12 : Outport  Port=16  OutDataType=sfix(16)  OutScaling=2^0
  Time Firing IO13 : Outport  Port=17  OutDataType=sfix(16)  OutScaling=2^0
  Time Firing IO14 : Outport  Port=18  OutDataType=sfix(16)  OutScaling=2^0
  Time Firing IO15 : Outport  Port=19  OutDataType=sfix(16)  OutScaling=2^0
  Time Firing IO16 : Outport  Port=20  OutDataType=sfix(16)  OutScaling=2^0
  Time Firing IO17 : Outport  Port=21  OutDataType=sfix(16)  OutScaling=2^0
  Time Firing IO18 : Outport  Port=22  OutDataType=sfix(16)  OutScaling=2^0
  Time Firing IO19 : Outport  Port=23  OutDataType=sfix(16)  OutScaling=2^0
  Time Firing IO20 : Outport  Port=24  OutDataType=sfix(16)  OutScaling=2^0
  Time Firing IO21 : Outport  Port=25  OutDataType=sfix(16)  OutScaling=2^0
  Time Firing IO22 : Outport  Port=26  OutDataType=sfix(16)  OutScaling=2^0
  Time Firing IO23 : Outport  Port=27  OutDataType=sfix(16)  OutScaling=2^0
  Time Firing IO24 : Outport  Port=28  OutDataType=sfix(16)  OutScaling=2^0
  Time Firing IO25 : Outport  Port=29  OutDataType=sfix(16)  OutScaling=2^0
  Time Firing IO26 : Outport  Port=30  OutDataType=sfix(16)  OutScaling=2^0
  Time Firing IO27 : Outport  Port=31  OutDataType=sfix(16)  OutScaling=2^0
  Time Firing IO28 : Outport  Port=32  OutDataType=sfix(16)  OutScaling=2^0
  Time Firing IO29 : Outport  Port=33  OutDataType=sfix(16)  OutScaling=2^0
  Time Firing IO30 : Outport  Port=34  OutDataType=sfix(16)  OutScaling=2^0
  Time Firing IO31 : Outport  Port=35  OutDataType=sfix(16)  OutScaling=2^0
  Time Firing IO32 : Outport  Port=36  OutDataType=sfix(16)  OutScaling=2^0
  Time Firing IO33 : Outport  Port=37  OutDataType=sfix(16)  OutScaling=2^0
  Time Firing IO34 : Outport  Port=38  OutDataType=sfix(16)  OutScaling=2^0
  Time Firing IO35 : Outport  Port=39  OutDataType=sfix(16)  OutScaling=2^0
  Time Firing IO36 : Outport  Port=40  OutDataType=sfix(16)  OutScaling=2^0
  Time Firing IO37 : Outport  Port=41  OutDataType=sfix(16)  OutScaling=2^0
  Time Firing IO38 : Outport  Port=42  OutDataType=sfix(16)  OutScaling=2^0
  Time Firing IO39 : Outport  Port=43  OutDataType=sfix(16)  OutScaling=2^0
  Time Firing IO40 : Outport  Port=44  OutDataType=sfix(16)  OutScaling=2^0
  Time Firing IO41 : Outport  Port=45  OutDataType=sfix(16)  OutScaling=2^0
  Time Firing IO42 : Outport  Port=46  OutDataType=sfix(16)  OutScaling=2^0
  Time Firing IO43 : Outport  Port=47  OutDataType=sfix(16)  OutScaling=2^0
  Time Firing IO44 : Outport  Port=48  OutDataType=sfix(16)  OutScaling=2^0
  Time Firing IO45 : Outport  Port=49  OutDataType=sfix(16)  OutScaling=2^0
  Time Firing IO46 : Outport  Port=50  OutDataType=sfix(16)  OutScaling=2^0
  Time Firing IO47 : Outport  Port=51  OutDataType=sfix(16)  OutScaling=2^0
  wires:
  Poisson1 IO/1(Time firing) -> bloque1 IO/1(Time Firing Poisson)
  Poisson1 IO/3(Time firing1) -> bloque1 IO1/1(Time Firing Poisson)
  " Max Torque Value Poisson1"/1 -> Poisson1 IO/1(" Max Torque Value ")
  Error Poisson1/1 -> Poisson1 IO/2(error)
  Poisson1 IO/2(I) -> Iout Poisson1/1
  " Max Torque Value Poisson2"/1 -> Poisson1 IO1/1(" Max Torque Value ")
  Error Poisson2/1 -> Poisson1 IO1/2(error)
  Poisson1 IO1/3(Time firing1) -> bloque1 IO3/1(Time Firing Poisson)
  bloque1 IO1/1(TimefiringIO0) -> Time Firing IO8/1
  bloque1 IO1/2(TimefiringIO1) -> Time Firing IO9/1
  bloque1 IO1/3(TimefiringIO2) -> Time Firing IO10/1
  bloque1 IO1/4(TimefiringIO3) -> Time Firing IO11/1
  bloque1 IO1/5(TimefiringIO4) -> Time Firing IO12/1
  bloque1 IO1/6(TimefiringIO5) -> Time Firing IO13/1
  bloque1 IO1/7(TimefiringIO6) -> Time Firing IO14/1
  bloque1 IO1/8(TimefiringIO7) -> Time Firing IO15/1
  bloque1 IO2/1(TimefiringIO0) -> Time Firing IO16/1
  bloque1 IO2/2(TimefiringIO1) -> Time Firing IO17/1
  bloque1 IO2/3(TimefiringIO2) -> Time Firing IO18/1
  bloque1 IO2/4(TimefiringIO3) -> Time Firing IO19/1
  bloque1 IO2/5(TimefiringIO4) -> Time Firing IO20/1
  bloque1 IO2/6(TimefiringIO5) -> Time Firing IO21/1
  bloque1 IO2/7(TimefiringIO6) -> Time Firing IO22/1
  bloque1 IO2/8(TimefiringIO7) -> Time Firing IO23/1
  bloque1 IO3/2(TimefiringIO1) -> Time Firing IO25/1
  bloque1 IO3/3(TimefiringIO2) -> Time Firing IO26/1
  bloque1 IO3/4(TimefiringIO3) -> Time Firing IO27/1
  bloque1 IO3/5(TimefiringIO4) -> Time Firing IO28/1
  bloque1 IO3/6(TimefiringIO5) -> Time Firing IO29/1
  bloque1 IO3/7(TimefiringIO6) -> Time Firing IO30/1
  bloque1 IO3/8(TimefiringIO7) -> Time Firing IO31/1
  bloque1 IO3/1(TimefiringIO0) -> Time Firing IO24/1
  " Max Torque Value Poisson3"/1 -> Poisson1 IO2/1(" Max Torque Value ")
  Error Poisson3/1 -> Poisson1 IO2/2(error)
  Poisson1 IO2/2(I) -> Iout Poisson3/1
  Poisson1 IO2/1(Time firing) -> bloque1 IO4/1(Time Firing Poisson)
  Poisson1 IO2/3(Time firing1) -> bloque1 IO5/1(Time Firing Poisson)
  bloque1 IO5/1(TimefiringIO0) -> Time Firing IO40/1
  bloque1 IO5/2(TimefiringIO1) -> Time Firing IO41/1
  bloque1 IO5/3(TimefiringIO2) -> Time Firing IO42/1
  bloque1 IO5/4(TimefiringIO3) -> Time Firing IO43/1
  bloque1 IO5/5(TimefiringIO4) -> Time Firing IO44/1
  bloque1 IO5/6(TimefiringIO5) -> Time Firing IO45/1
  bloque1 IO5/7(TimefiringIO6) -> Time Firing IO46/1
  bloque1 IO5/8(TimefiringIO7) -> Time Firing IO47/1
  Poisson1 IO1/2(I) -> Iout Poisson2/1
  Poisson1 IO1/1(Time firing) -> bloque1 IO2/1(Time Firing Poisson)
  bloque1 IO/1(TimefiringIO0) -> Time Firing IO0/1
  bloque1 IO/2(TimefiringIO1) -> Time Firing IO1/1
  bloque1 IO/3(TimefiringIO2) -> Time Firing IO2/1
  bloque1 IO/4(TimefiringIO3) -> Time Firing IO3/1
  bloque1 IO/5(TimefiringIO4) -> Time Firing IO4/1
  bloque1 IO/6(TimefiringIO5) -> Time Firing IO5/1
  bloque1 IO/7(TimefiringIO6) -> Time Firing IO6/1
  bloque1 IO/8(TimefiringIO7) -> Time Firing IO7/1
  bloque1 IO4/1(TimefiringIO0) -> Time Firing IO32/1
  bloque1 IO4/2(TimefiringIO1) -> Time Firing IO33/1
  bloque1 IO4/3(TimefiringIO2) -> Time Firing IO34/1
  bloque1 IO4/4(TimefiringIO3) -> Time Firing IO35/1
  bloque1 IO4/5(TimefiringIO4) -> Time Firing IO36/1
  bloque1 IO4/6(TimefiringIO5) -> Time Firing IO37/1
  bloque1 IO4/7(TimefiringIO6) -> Time Firing IO38/1
  bloque1 IO4/8(TimefiringIO7) -> Time Firing IO39/1

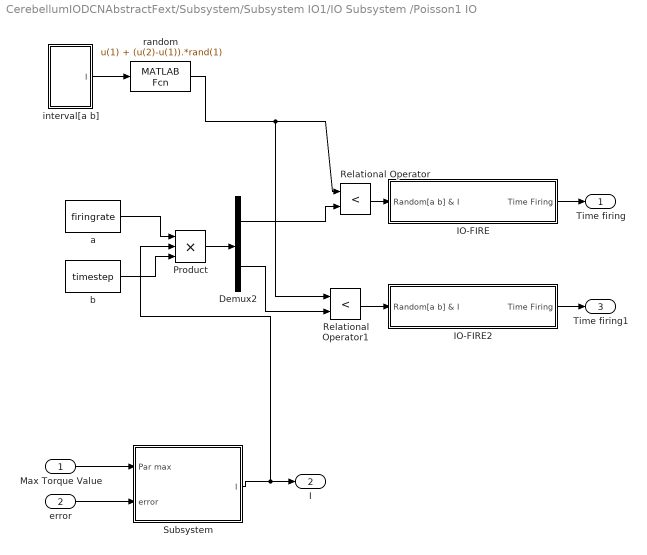
== system CerebellumIODCNAbstractFext/Subsystem/Subsystem IO1/IO Subsystem /Poisson1 IO ==
  " Max Torque Value " : Inport  OutDataType=sfix(16)  OutScaling=2^0
  error : Inport  Port=2  OutDataType=sfix(16)  OutScaling=2^0
  Demux2 : Demux  Outputs=2
  IO-FIRE : Subsystem
  IO-FIRE2 : Subsystem
  Product : Product  Inputs=3  OutDataType=sfix(16)  OutScaling=2^0  RndMeth=Zero
  Relational Operator : RelationalOperator  Operator=<  LogicOutDataTypeMode=boolean  LogicDataType=sint(32)  OutDataTypeStr=boolean
  Relational Operator1 : RelationalOperator  Operator=<  LogicOutDataTypeMode=boolean  LogicDataType=sint(32)  OutDataTypeStr=boolean
  Subsystem : Subsystem
  a : Constant  Value=firingrate  OutDataType=sfix(16)  OutScaling=2^0
  b : Constant  Value=timestep  OutDataType=sfix(16)  OutScaling=2^0
  interval[a b] : Subsystem
  random : MATLABFcn  MATLABFcn=u(1) + (u(2)-u(1)).*rand(1)
  Time firing : Outport  OutDataType=sfix(16)  OutScaling=2^0
  I : Outport  Port=2  OutDataType=sfix(16)  OutScaling=2^0
  Time firing1 : Outport  Port=3  OutDataType=sfix(16)  OutScaling=2^0
  wires:
  interval[a b]/1(I) -> random/1
  " Max Torque Value "/1 -> Subsystem/1(Par max)
  error/1 -> Subsystem/2(error)
  Subsystem/1(I) -> I/1, Product/2
  Demux2/1 -> Relational Operator/2
  Demux2/2 -> Relational Operator1/2
  a/1 -> Product/1
  Relational Operator/1 -> IO-FIRE/1(Random[a b] & I)
  IO-FIRE/1(Time Firing) -> Time firing/1
  Relational Operator1/1 -> IO-FIRE2/1(Random[a b] & I)
  Product/1 -> Demux2/1
  b/1 -> Product/3
  random/1 -> Relational Operator/1, Relational Operator1/1
  IO-FIRE2/1(Time Firing) -> Time firing1/1

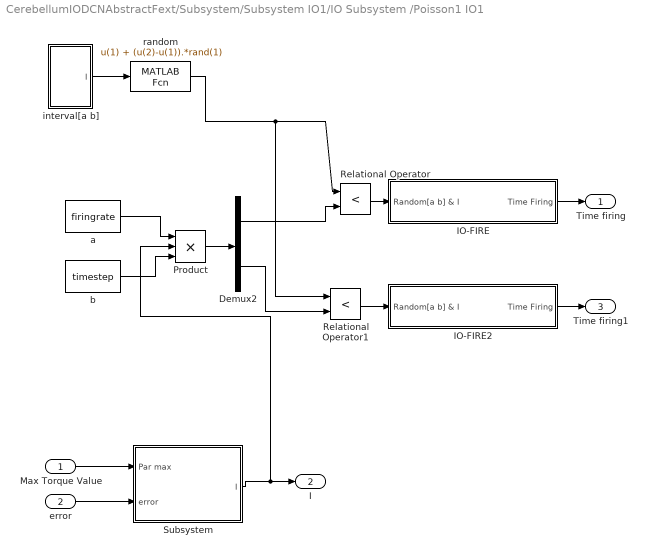
== system CerebellumIODCNAbstractFext/Subsystem/Subsystem IO1/IO Subsystem /Poisson1 IO1 ==
  " Max Torque Value " : Inport  OutDataType=sfix(16)  OutScaling=2^0
  error : Inport  Port=2  OutDataType=sfix(16)  OutScaling=2^0
  Demux2 : Demux  Outputs=2
  IO-FIRE : Subsystem
  IO-FIRE2 : Subsystem
  Product : Product  Inputs=3  OutDataType=sfix(16)  OutScaling=2^0  RndMeth=Zero
  Relational Operator : RelationalOperator  Operator=<  LogicOutDataTypeMode=boolean  LogicDataType=sint(32)  OutDataTypeStr=boolean
  Relational Operator1 : RelationalOperator  Operator=<  LogicOutDataTypeMode=boolean  LogicDataType=sint(32)  OutDataTypeStr=boolean
  Subsystem : Subsystem
  a : Constant  Value=firingrate  OutDataType=sfix(16)  OutScaling=2^0
  b : Constant  Value=timestep  OutDataType=sfix(16)  OutScaling=2^0
  interval[a b] : Subsystem
  random : MATLABFcn  MATLABFcn=u(1) + (u(2)-u(1)).*rand(1)
  Time firing : Outport  OutDataType=sfix(16)  OutScaling=2^0
  I : Outport  Port=2  OutDataType=sfix(16)  OutScaling=2^0
  Time firing1 : Outport  Port=3  OutDataType=sfix(16)  OutScaling=2^0
  wires:
  interval[a b]/1(I) -> random/1
  " Max Torque Value "/1 -> Subsystem/1(Par max)
  error/1 -> Subsystem/2(error)
  Subsystem/1(I) -> I/1, Product/2
  Demux2/1 -> Relational Operator/2
  Demux2/2 -> Relational Operator1/2
  a/1 -> Product/1
  Relational Operator/1 -> IO-FIRE/1(Random[a b] & I)
  IO-FIRE/1(Time Firing) -> Time firing/1
  Relational Operator1/1 -> IO-FIRE2/1(Random[a b] & I)
  Product/1 -> Demux2/1
  b/1 -> Product/3
  random/1 -> Relational Operator/1, Relational Operator1/1
  IO-FIRE2/1(Time Firing) -> Time firing1/1

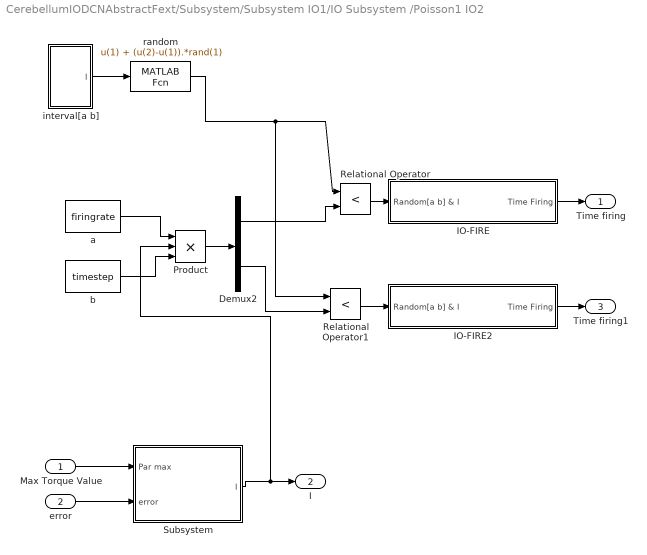
== system CerebellumIODCNAbstractFext/Subsystem/Subsystem IO1/IO Subsystem /Poisson1 IO2 ==
  " Max Torque Value " : Inport  OutDataType=sfix(16)  OutScaling=2^0
  error : Inport  Port=2  OutDataType=sfix(16)  OutScaling=2^0
  Demux2 : Demux  Outputs=2
  IO-FIRE : Subsystem
  IO-FIRE2 : Subsystem
  Product : Product  Inputs=3  OutDataType=sfix(16)  OutScaling=2^0  RndMeth=Zero
  Relational Operator : RelationalOperator  Operator=<  LogicOutDataTypeMode=boolean  LogicDataType=sint(32)  OutDataTypeStr=boolean
  Relational Operator1 : RelationalOperator  Operator=<  LogicOutDataTypeMode=boolean  LogicDataType=sint(32)  OutDataTypeStr=boolean
  Subsystem : Subsystem
  a : Constant  Value=firingrate  OutDataType=sfix(16)  OutScaling=2^0
  b : Constant  Value=timestep  OutDataType=sfix(16)  OutScaling=2^0
  interval[a b] : Subsystem
  random : MATLABFcn  MATLABFcn=u(1) + (u(2)-u(1)).*rand(1)
  Time firing : Outport  OutDataType=sfix(16)  OutScaling=2^0
  I : Outport  Port=2  OutDataType=sfix(16)  OutScaling=2^0
  Time firing1 : Outport  Port=3  OutDataType=sfix(16)  OutScaling=2^0
  wires:
  interval[a b]/1(I) -> random/1
  " Max Torque Value "/1 -> Subsystem/1(Par max)
  error/1 -> Subsystem/2(error)
  Subsystem/1(I) -> I/1, Product/2
  Demux2/1 -> Relational Operator/2
  Demux2/2 -> Relational Operator1/2
  a/1 -> Product/1
  Relational Operator/1 -> IO-FIRE/1(Random[a b] & I)
  IO-FIRE/1(Time Firing) -> Time firing/1
  Relational Operator1/1 -> IO-FIRE2/1(Random[a b] & I)
  Product/1 -> Demux2/1
  b/1 -> Product/3
  random/1 -> Relational Operator/1, Relational Operator1/1
  IO-FIRE2/1(Time Firing) -> Time firing1/1

== system CerebellumIODCNAbstractFext/Subsystem/Subsystem IO1/IO Subsystem /bloque1 IO ==
  Time Firing Poisson : Inport  OutDataType=sfix(16)  OutScaling=2^0
  TimefiringIO0 : Outport  OutDataType=sfix(16)  OutScaling=2^0
  TimefiringIO1 : Outport  Port=2  OutDataType=sfix(16)  OutScaling=2^0
  TimefiringIO2 : Outport  Port=3  OutDataType=sfix(16)  OutScaling=2^0
  TimefiringIO3 : Outport  Port=4  OutDataType=sfix(16)  OutScaling=2^0
  TimefiringIO4 : Outport  Port=5  OutDataType=sfix(16)  OutScaling=2^0
  TimefiringIO5 : Outport  Port=6  OutDataType=sfix(16)  OutScaling=2^0
  TimefiringIO6 : Outport  Port=7  OutDataType=sfix(16)  OutScaling=2^0
  TimefiringIO7 : Outport  Port=8  OutDataType=sfix(16)  OutScaling=2^0
  wires:
  Time Firing Poisson/1 -> TimefiringIO0/1, TimefiringIO1/1, TimefiringIO2/1, TimefiringIO3/1, TimefiringIO4/1, TimefiringIO5/1, TimefiringIO6/1, TimefiringIO7/1

== system CerebellumIODCNAbstractFext/Subsystem/Subsystem IO1/IO Subsystem /bloque1 IO1 ==
  Time Firing Poisson : Inport  OutDataType=sfix(16)  OutScaling=2^0
  TimefiringIO0 : Outport  OutDataType=sfix(16)  OutScaling=2^0
  TimefiringIO1 : Outport  Port=2  OutDataType=sfix(16)  OutScaling=2^0
  TimefiringIO2 : Outport  Port=3  OutDataType=sfix(16)  OutScaling=2^0
  TimefiringIO3 : Outport  Port=4  OutDataType=sfix(16)  OutScaling=2^0
  TimefiringIO4 : Outport  Port=5  OutDataType=sfix(16)  OutScaling=2^0
  TimefiringIO5 : Outport  Port=6  OutDataType=sfix(16)  OutScaling=2^0
  TimefiringIO6 : Outport  Port=7  OutDataType=sfix(16)  OutScaling=2^0
  TimefiringIO7 : Outport  Port=8  OutDataType=sfix(16)  OutScaling=2^0
  wires:
  Time Firing Poisson/1 -> TimefiringIO2/1, TimefiringIO0/1, TimefiringIO1/1, TimefiringIO3/1, TimefiringIO4/1, TimefiringIO5/1, TimefiringIO7/1, TimefiringIO6/1

== system CerebellumIODCNAbstractFext/Subsystem/Subsystem IO1/IO Subsystem /bloque1 IO2 ==
  Time Firing Poisson : Inport  OutDataType=sfix(16)  OutScaling=2^0
  TimefiringIO0 : Outport  OutDataType=sfix(16)  OutScaling=2^0
  TimefiringIO1 : Outport  Port=2  OutDataType=sfix(16)  OutScaling=2^0
  TimefiringIO2 : Outport  Port=3  OutDataType=sfix(16)  OutScaling=2^0
  TimefiringIO3 : Outport  Port=4  OutDataType=sfix(16)  OutScaling=2^0
  TimefiringIO4 : Outport  Port=5  OutDataType=sfix(16)  OutScaling=2^0
  TimefiringIO5 : Outport  Port=6  OutDataType=sfix(16)  OutScaling=2^0
  TimefiringIO6 : Outport  Port=7  OutDataType=sfix(16)  OutScaling=2^0
  TimefiringIO7 : Outport  Port=8  OutDataType=sfix(16)  OutScaling=2^0
  wires:
  Time Firing Poisson/1 -> TimefiringIO0/1, TimefiringIO1/1, TimefiringIO2/1, TimefiringIO3/1, TimefiringIO4/1, TimefiringIO5/1, TimefiringIO6/1, TimefiringIO7/1
